simulink model "SampleTime"  (Simulink 10.1)
settings: Solver=ode45  StartTime=0.0  StopTime=9.82  RelTol=1e-3
settings Model: Creator=iba  LastModifiedBy=iba
settings DataIOCC: SaveFormat=Dataset  ReturnWorkspaceOutputs=on
settings OptimizationCC: LifeSpan=auto
settings DebuggingCC: UnderspecifiedInitializationDetection=Simplified  MergeDetectMultiDrivingBlocksExec=error  SFUnexpectedBacktrackingDiag=error  SFNoUnconditionalDefaultTransitionDiag=error  SFExecutionAtInitializationDiag=warning  ArithmeticOperatorsInVariantConditions=error
settings HardwareCC: ProdBitPerPointer=64  ProdBitPerSizeT=64  ProdBitPerPtrDiffT=64  ProdLargestAtomicFloat=Float  ProdIntDivRoundTo=Zero  ProdEndianess=LittleEndian  ProdWordSize=64  ProdHWDeviceType=Intel->x86-64 (Windows64)
settings ModelReferenceCC: PropagateSignalLabelsOutOfModel=on
settings SFSimCC: SimUseLocalCustomCode=on  CustomCodeUndefinedFunction=FilterOut
settings RTWCC: RTWUseLocalCustomCode=on
settings CodeAppCC: StateflowObjectComments=off
settings GRTTargetCC: TargetLangStandard=C99 (ISO)  CombineOutputUpdateFcns=on  GRTInterface=off
settings ConfigComp: CovMetricSettings=dwe  CovHtmlReporting=off  CovSaveCumulativeToWorkspaceVar=off  CovSaveSingleToWorkspaceVar=off  CovExternalEMLEnable=on

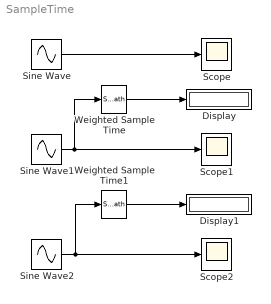
== system SampleTime ==
  Display : Display
  Display1 : Display
  Scope : Scope
  Scope1 : Scope
  Scope2 : Scope
  Sine Wave : Sin  SampleTime=0
  Sine Wave1 : Sin  SampleTime=1
  Sine Wave2 : Sin  SampleTime=2
  Weighted Sample Time : SampleTimeMath  TsampMathOp=Ts Only
  Weighted Sample Time1 : SampleTimeMath  TsampMathOp=Ts Only
  wires:
  Sine Wave/1 -> Scope/1
  Sine Wave1/1 -> Scope1/1, Weighted Sample Time/1
  Weighted Sample Time/1 -> Display/1
  Weighted Sample Time1/1 -> Display1/1
  Sine Wave2/1 -> Weighted Sample Time1/1, Scope2/1
